simulink model "BPSK____RECEIVER____REAL_TIME"  (R2022a)
settings: Solver=VariableStepAuto  StartTime=0.0  StopTime=inf  RelTol=1e-3
undefined symbols (not defined in the file or in its folder): designMultirateFIR, Fs, ip, usb
libraries: commsync2 x2, commfilt2 x2, dspsrcs4 x2, plutoradiolib x1, commrfcorlib x1, commdigbbndpm3 x1, dsparch4 x1, dspmlti4 x1, sdrrlib x1, simulink x1
settings Model: Creator=Nithish  LastModifiedBy=Nithish

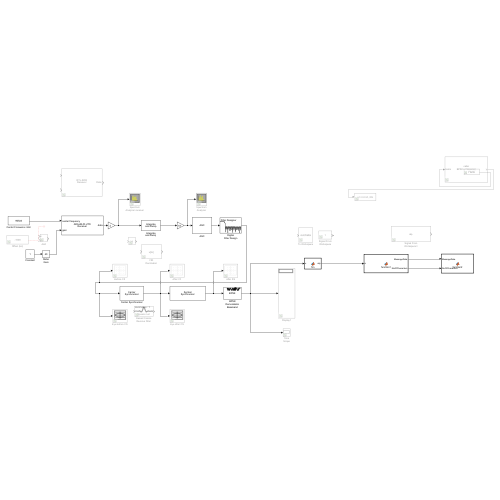
[thumbnail: Simulink's stored preview of the top-level diagram]
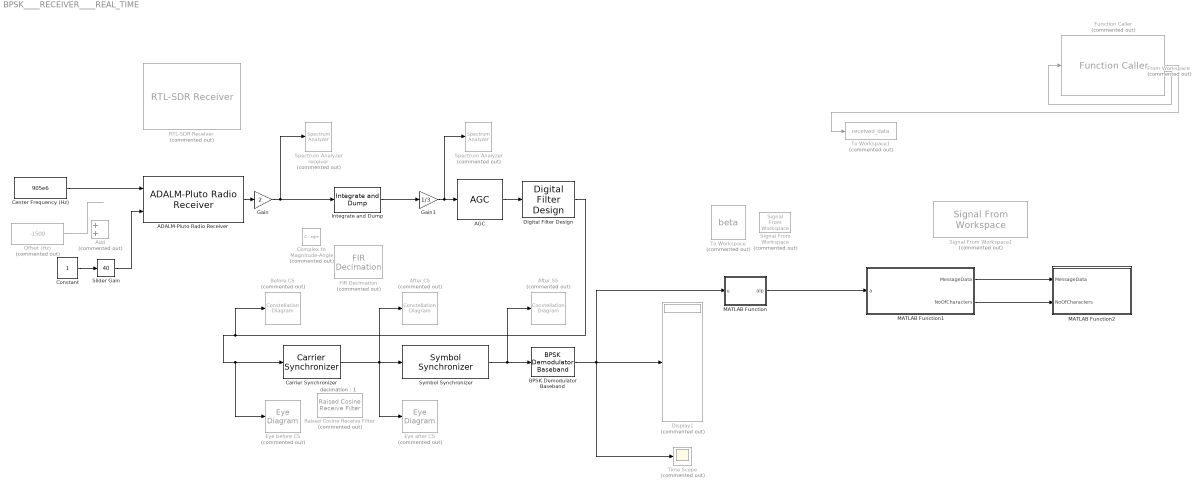
== system BPSK____RECEIVER____REAL_TIME ==
  note: decimation : 1
  ADALM-Pluto Radio Receiver : plutoradiolib/ADALM-Pluto Radio Receiver  RadioID=usb:0  uri=ip:10.0.0.200  CenterFrequencySource=Input Port  CenterFrequency=2.4e9  GainSource=AGC Slow Attack  GainSourceBlock=Input Port  Gain=10  ChannelMapping=1  BasebandSampleRate=240e3  OutputDataType=single  SamplesPerFrame=300000  OverflowOutputPort=off  EnableBurstMode=off  NumFramesInBurst=1  ShowAdvancedProperties=off  UseCustomFilter=off  filtPathRates=[737280000 11520000 3840000 1920000 960000 240000]  filtCoefficients=[-192 82 85 -215 228 -102 -110 290 -318 145 160 -426 471 -215 -238 633 -697 318 349 -923 1009 -457 -498 1309 -1423 640 693 -1812 1959 -876 -945 2458 -2647 1180 1268 -3290 3534 -1572 -1688 4375 -4698 2091 2247 -5836 6284 -2807 -3031 7918 -8588 3870 4225 -11182 12324 -5662 -6330 17255 -19735 9507 11312 -33568 43355 -25227 -42139 305542 305542 -42139 -25227 43355 -33568 11312 9507 -19735 17255 -6330 -5662 12324 -11182 4225 3870 -8588 7918 -3031 -2807 6284 -5836 2247 2091 -4698 4375 -1688 -1572 3534 -3290 1268 1180 -2647 2458 -945 -876 1959 -1812 693 640 -1423 1309 -498 -457 1009 -923 349 318 -697 633 -238 -215 471 -426 160 145 -318 290 -110 -102 228 -215 85 82 -192]  filtCoefficientSize=128  filtDecimInterpFactor=4  filtGain=-12  filtRFBandwidth=18000000  filterConfigStruct=struct()  EnableQuadratureCorrection=on  EnableRFDCCorrection=on  EnableBasebandDCCorrection=on  FrequencyCorrection=0  OverrideSampleTime=off  SampleTime=0.02  DataTimeout=Inf  ENSMPinControlMode=None  BISTLoopbackMode=Disabled  BISTToneInject=Disabled  BISTSignalGen=PRBS  BISTToneFreq=Fs/32  BISTToneLevel=0
      settings: SourceProductBaseCode=PLUTO
  AGC : commrfcorlib/AGC  LegacyMode=off  DetectorMethod=Rectifier  LoopMethod=Linear  UpdatePeriod=100  StepSize=0.1  AdaptationStepSize=0.1  DesiredOutputPower=.1  AveragingLength=100  MaximumGain=30  MaxPowerGain=50  GainOutputPort=off  InputPowerOutputPort=off  SimulateUsing=Interpreted execution
  Add : Sum  Commented=on
  After CS : ConstellationDiagram  Commented=on  WindowPosition=[445.000000,24.000000,341.000000,346.000000,]  ScopeFrameLocation=window  SamplesPerSymbol=10  SymbolsToDisplaySource=Property  SymbolsToDisplay=100  ReferenceConstellation=BPSK  XLimits=[-1.8347 1.888]  YLimits=[-1.8347 1.888]  DefaultConfigurationName=comm.scopes.ConstellationDiagramBlockCfg
  After SS : ConstellationDiagram  Commented=on  WindowPosition=[807.000000,406.000000,341.000000,345.000000,]  ScopeFrameLocation=window  SamplesPerSymbol=10  SymbolsToDisplaySource=Property  SymbolsToDisplay=200  ReferenceConstellation=BPSK  XLimits=[-1.3383 1.3452]  YLimits=[-1.3383 1.3452]  DefaultConfigurationName=comm.scopes.ConstellationDiagramBlockCfg
  BPSK Demodulator Baseband : commdigbbndpm3/BPSK Demodulator Baseband  DecType=Hard decision  VarSource=Dialog  Variance=1  Ph=0  outDtype=Inherit via internal rule  derotateFactorWordLen=16  derotateFactorDataTypeStr=Inherit: Same word length as input  derotateFactorLastDataTypeStr=Inherit: Same word length as input
  Before CS : ConstellationDiagram  Commented=on  WindowPosition=[92.000000,21.000000,342.000000,346.000000,]  ScopeFrameLocation=window  SamplesPerSymbol=30  SymbolsToDisplaySource=Property  SymbolsToDisplay=100  ReferenceConstellation=BPSK  XLimits=[-1.5991 1.3577]  YLimits=[-1.9686 1.7273]  DefaultConfigurationName=comm.scopes.ConstellationDiagramBlockCfg
  Carrier Synchronizer : commsync2/Carrier Synchronizer  Modulation=BPSK  ModulationPhaseOffset=Auto  CustomPhaseOffset=pi/4  SamplesPerSymbol=4  DampingFactor=0.707  NormalizedLoopBandwidth=.01  EstimatedPhaseErrorOutputPort=off  SimulateUsing=Code generation
  Center Frequency (Hz) : Constant  Value=905e6
  Complex to Magnitude-Angle : ComplexToMagnitudeAngle  Commented=on  Output=Magnitude
  Constant : Constant
  Digital Filter Design : dsparch4/Digital Filter Design  mwdsp_browser_bugfix_var=off
  Display1 : Display  Commented=on
  Eye after CS : EyeDiagram  Commented=on
  Eye before CS : EyeDiagram  Commented=on
  FIR Decimation : dspmlti4/FIR Decimation  Commented=on  FilterSource=Auto  h=designMultirateFIR(1,2)  D=3  filtStruct=Direct form  FilterObject=FDECIM  InputProcessing=Columns as channels (frame based)  framing=Enforce single-rate processing  inputOffset=0  outputBufInitCond=0  roundingMode=Floor  overflowMode=off  firstCoeffDataTypeStr=Inherit: Same word length as input  firstCoeffMin=[]  firstCoeffMax=[]  firstCoeffLastDataTypeStr=Inherit: Same word length as input  outputDataTypeStr=Inherit: Same as accumulator  outputMin=[]  outputMax=[]  outputLastDataTypeStr=Inherit: Same as accumulator
  From Workspace : FromWorkspace  Commented=on  VariableName=Hello
  Function Caller : FunctionCaller  Commented=on  FunctionPrototype=y = BPSKworkspace(Hello)  InputArgumentSpecifications=<Enter example>  OutputArgumentSpecifications=<Enter example>
  Gain : Gain  Gain=2
  Gain1 : Gain  Gain=1/3
  Integrate and Dump : commfilt2/Integrate and Dump  obssamples=3  offsetsamples=0  nodump=off  roundingMode=Floor  overflowMode=off  outputDataTypeStr=Inherit: Same as accumulator  outputLastDataTypeStr=Inherit: Same as accumulator
  MATLAB Function : MATLAB Function  TreatAsAtomicUnit=on
  MATLAB Function1 : MATLAB Function  TreatAsAtomicUnit=on
  MATLAB Function2 : MATLAB Function  TreatAsAtomicUnit=on
  Offset (Hz) : Constant  Commented=on  Value=-1500
  RTL-SDR Receiver : sdrrlib/RTL-SDR Receiver  Commented=on  IPAddress=0  CenterFrequencySource=Input port  CenterFrequency=102.5e6  GainSource=Input port  Gain=0  ADCRate=240e3  FrequencyCorrection=0  LostSamplesOutputPort=off  LatencyOutputPort=off  OutputDataType=single  FrameLength=3000  EnableBurstMode=off  NumFramesInBurst=20  sobjType=sdrr.internal.SDRRTLReceiverSL  dataUDPPort=-1  ctrlUDPPort=-1  subDeviceList=nosubdev  sdrBlockType=SDRBlockTypeSLT.SDRRxBlock  requester=UNUSED_BY_SFCN  sdrExecutionMode=SDRExecutionModeSLT.ExecModeHW  BypassUserLogic=off  DecimatorSelect=DDC decimator  SourceSelect=RF data  SineAmplitude=16000  EnableInternalClock=off  BypassIQBalance=off  IFBandwidth=40e6  ADCRateSource=Dialog  IntermediateFrequency=0  DecimationFactorSource=Dialog  DecimationFactor=512  RFFrequencyIsTunable=logical(1)  SampleTime=(3000)/(240e3)  IFBandwidthSource=Dialog  SineFrequency=30000  BypassDCBlockingFilter=off  IntermediateFrequencySource=Dialog  IQBalanceCoefficients=64  SkipAllHardwareResetAndInitialization=off  EnableIQCalibrationTable=on  CacheIQCalibrationTable=off  EnableOffsetTuning=off  EnableRTLAGC=off  EnableTestMode=off  EnableTunerAGC=off  FrequencyCorrectionSource=Dialog  NumMLBuffers=128  NumUSBBuffers=16  RTLCrystalFrequency=28800000  TunerCrystalFrequency=28800000
      settings: SourceProductBaseCode=RTLSDR
  Raised Cosine Receive Filter : commfilt2/Raised Cosine Receive Filter  Commented=on  filtType=Square root  R=.5  filtSpan=4  N=10  downFactor=1  downOffset=0  filterGain=1  InputProcessing=Columns as channels (frame based)  RateOptions=Enforce single-rate processing  framing=Mute  checkCoeff=off  variableName=rcRxFilt1  currentFiltSpan=4  D=(4)/2  inputOffset=0  sampMode=Mute  saveAsFlag=0  rateMode=Downsampling  checkGain=Normalized  launchFVT=on  roundingMode=Floor  overflowMode=off  coeffDataTypeStr=Inherit: Same word length as input  coeffMin=[]  coeffMax=[]  coeffLastDataTypeStr=Inherit: Same word length as input  accumDataTypeStr=Inherit: Same as product output  accumLastDataTypeStr=Inherit: Same as product output  outputDataTypeStr=Inherit: Same as accumulator  outputMin=[]  outputMax=[]  outputLastDataTypeStr=Inherit: Same as accumulator
  Signal From Workspace : dspsrcs4/Signal From Workspace  Commented=on  X=1  Ts=4  nsamps=1  OutputAfterFinalValue=Setting to zero  ignoreOrWarnInputAndFrameLengths=off  OutputFrames=off
  Signal From Workspace1 : dspsrcs4/Signal From Workspace  Commented=on  X=alp  Ts=5  nsamps=10000  OutputAfterFinalValue=Setting to zero  ignoreOrWarnInputAndFrameLengths=off  OutputFrames=off
  Slider Gain : simulink/Math Operations/Slider Gain  gain=40  low=5  high=60
  Spectrum Analyzer : SpectrumAnalyzer  Commented=on
  Spectrum Analyzer receiver : SpectrumAnalyzer  Commented=on
  Symbol Synchronizer : commsync2/Symbol Synchronizer  Modulation=PAM/PSK/QAM  TimingErrorDetector=Mueller-Muller (decision-directed)  SamplesPerSymbol=10  DampingFactor=1  NormalizedLoopBandwidth=0.01  DetectorGain=2.7  TimingErrorOutputPort=off  SimulateUsing=Code generation
      settings: SourceProductBaseCode=CM
  Time Scope : Scope  Commented=on
  To Workspace : ToWorkspace  Commented=on  VariableName=beta  SaveFormat=Structure  SampleTime=-1
      settings: Save2DSignal=2-D array (concatenate along first dimension)
  To Workspace1 : ToWorkspace  Commented=on  VariableName=received_data  SaveFormat=Structure  SampleTime=-1
      settings: Save2DSignal=2-D array (concatenate along first dimension)
  wires:
  Offset (Hz)/1 -> ?
  Function Caller/1 -> To Workspace1/1
  Constant/1 -> Slider Gain/1
  Digital Filter Design/1 -> Before CS/1, Eye before CS/1, Carrier Synchronizer/1
  Gain1/1 -> Spectrum Analyzer/1, AGC/1
  ADALM-Pluto Radio Receiver/1 -> Gain/1
  AGC/1 -> Digital Filter Design/1
  Gain/1 -> Integrate and Dump/1, Spectrum Analyzer receiver/1
  Symbol Synchronizer/1 -> BPSK Demodulator Baseband/1, After SS/1
  Center Frequency (Hz)/1 -> ADALM-Pluto Radio Receiver/1
  Slider Gain/1 -> ADALM-Pluto Radio Receiver/2
  Integrate and Dump/1 -> Gain1/1
  From Workspace/1 -> Function Caller/1
  Carrier Synchronizer/1 -> Symbol Synchronizer/1, Eye after CS/1, After CS/1
  MATLAB Function1/2(NoOfCharacters) -> MATLAB Function2/2(NoOfCharacters)
  MATLAB Function1/1(MessageData) -> MATLAB Function2/1(MessageData)
  BPSK Demodulator Baseband/1 -> MATLAB Function/1(u), Display1/1, Time Scope/1
  MATLAB Function/1(alp) -> MATLAB Function1/1(a)

== matlab function BPSK____RECEIVER____REAL_TIME/MATLAB Function1 ==
  data: a input; MessageData output size=[5000,5000] [-10000000..100000000000]; NoOfCharacters output
function [MessageData,NoOfCharacters] =  function1(a)

zen = a ;

prb = [0 0 0 0 1 1 1 1 0 0 0 0 1 1 1 1]';

prbdet = comm.PreambleDetector(prb,'Input','Bit');

idx = prbdet(zen);

MessageData = zen((idx(1)+1):(idx(2)-16)).';

NoOfCharacters = size(MessageData,2)/8;

%reshape(c, 8,(idx(4)+1):((idx(5)-16)/8)).';

== matlab function BPSK____RECEIVER____REAL_TIME/MATLAB Function ==
  data: u input; alp output
function alp = fcn(u)
%Hell = out.beta.signals.values;
alp = u(1:10000,1,1);

== matlab function BPSK____RECEIVER____REAL_TIME/MATLAB Function2 ==
  data: MessageData input; NoOfCharacters input
function function2(MessageData,NoOfCharacters)

%leo 

turtle = reshape(MessageData,8,NoOfCharacters).';

%snake = zeros(raph,8)

%for i = 1:raph
 %   for j = 1:8
   %     snake(i,j) = turtle(i,j)
  %  end
%end   

%rabbit = snake(1,1:8)
%eagle = rabbit
%sprintf('%e',turtle)

value = 0;
array = zeros(1,NoOfCharacters);
class(value);
for k = 1:NoOfCharacters
    for l = 1:8
        value = value + double(turtle(k,9-l)*2^(l-1));
    end
    array(k) = value;
    value = 0;
end   

a = char(array);

%type(a)

fprintf('%s',a)

return
